simulink model "FIR_32tap"  (Simulink 7.0)
settings: Solver=FixedStepDiscrete  StartTime=0.0  StopTime=2048*sample_time  RelTol=1e-3
PreLoadFcn:
  | FIR_32tap_setup
InitFcn:
  | %% DSPBuilder Start
  | alt_dspbuilder_update_model(bdroot)
  | %% DSPBuilder End
undefined symbols (not defined in the file): fir_coeff, get, sample_time
libraries: allblocks_alteradspbuilder2 x43, dspsnks4 x2, Stratix_EP2S60_alteradspbuilder2 x2
settings Model: Creator=davlin  LastModifiedBy=davlin
settings DebuggingCC: SaveWithParameterizedLinksMsg=none
settings GRTTargetCC: TargetFcnLib=ansi_tfl_tmw.mat

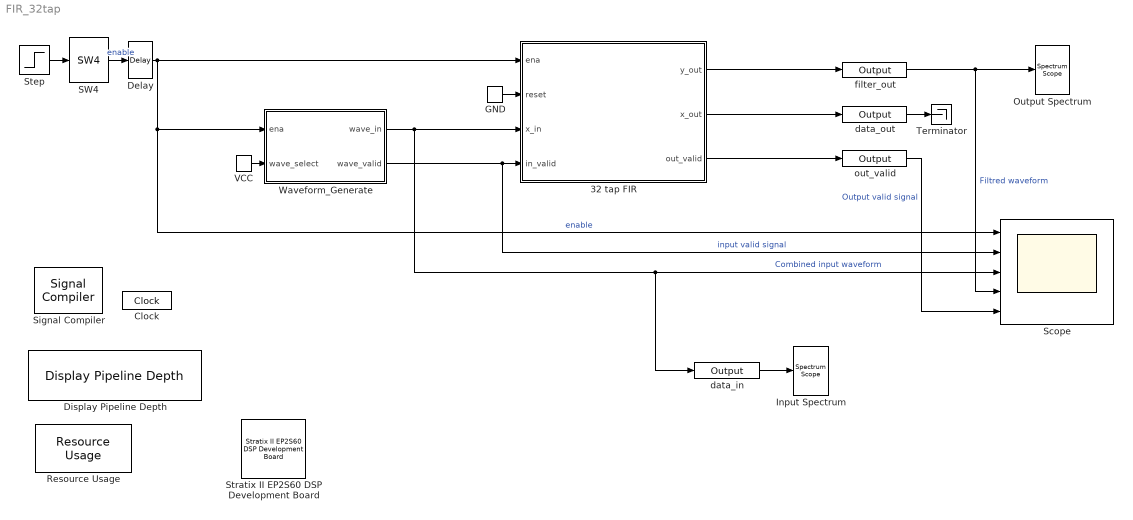
== system FIR_32tap ==
  32 tap FIR : Subsystem
  Clock : allblocks_alteradspbuilder2/Clock  ClockPeriod=clock_period  ClockPeriodUnit=ns  SampleTime=sample_time  SimulationStartCycle=5  PhaseOffset=0  Reset=aclr  ResetType=Active Low  Export=off
  Delay : allblocks_alteradspbuilder2/Delay  pipeline=1  pipeline_display=1  ClockPhase=1  use_ena=off  use_sclr=off  allowFloatingPointOverride=on  logOutputs=off  logFile=C:\Training\DSP_Training\Labs\DSPB_QII_V_9_0\Ex3\partc\tb_FIR_32tap\FIR%5F32tap_Delay.fixedpointlog  use_init=off  reset_value=1
  Display Pipeline Depth : allblocks_alteradspbuilder2/Display Pipeline Depth  DisplayLatencyOnBlocks=on
  GND : allblocks_alteradspbuilder2/GND  SpecifyClock=on  clock=Clock
  Input Spectrum : dspsnks4/Spectrum Scope  DialogController=dspdialog.SpectrumScope  DialogControllerArgs=DataTag0  SystemSampleTime=-1  ScopeProperties=on  Domain=Frequency  HorizSpan=1  UseBuffer=on  BufferSize=128  Overlap=64  inpFftLenInherit=off  FFTlength=128  numAvg=2  DisplayProperties=off  AxisGrid=on  Memory=off  FrameNumber=on  AxisLegend=off  AxisZoom=off  OpenScopeAtSimStart=on  OpenScopeImmediately=off  FigPos=get(0,'defaultfigureposition')  AxisProperties=off  XUnits=Hertz  XRange=[0...Fs/2]  InheritXIncr=on  XIncr=1.0  XLabel=Samples  XLimit=Auto  YUnits=dB  XMax=1  XMin=0  YLabel=Magnitude-squared, dB  LineProperties=off  wintypeSpecScope=Kaiser  RsSpecScope=50  betaSpecScope=5  winsampSpecScope=Periodic
      settings: YMin=1.0709621458062  YMax=69.4519012654706
  Output Spectrum : dspsnks4/Spectrum Scope  DialogController=dspdialog.SpectrumScope  DialogControllerArgs=DataTag1  SystemSampleTime=-1  ScopeProperties=on  Domain=Frequency  HorizSpan=1  UseBuffer=on  BufferSize=128  Overlap=64  inpFftLenInherit=off  FFTlength=128  numAvg=2  DisplayProperties=off  AxisGrid=on  Memory=off  FrameNumber=on  AxisLegend=off  AxisZoom=off  OpenScopeAtSimStart=on  OpenScopeImmediately=off  FigPos=get(0,'defaultfigureposition')  AxisProperties=off  XUnits=Hertz  XRange=[0...Fs/2]  InheritXIncr=on  XIncr=1.0  XLabel=Samples  XLimit=Auto  YUnits=dB  XMax=1  XMin=0  YLabel=Magnitude-squared, dB  LineProperties=off  wintypeSpecScope=Kaiser  RsSpecScope=50  betaSpecScope=5  winsampSpecScope=Periodic
      settings: YMin=-2.30591385737013  YMax=68.9595708716215
  Resource Usage : allblocks_alteradspbuilder2/Resource Usage  logic=3 %%  memory=< 1 %%  dsp=11 %%  memoryLable=Block RAM  dspLable=DSP
  SW4 : Stratix_EP2S60_alteradspbuilder2/SW4  iofile=C:\Training\DSP_Training\Labs\DSPB_QII_V_9_0\Ex3\partc\tb_FIR_32tap\FIR%5F32tap_SW4.salt  externalType=Inferred  SpecifyClock=on  clock=Clock  location=Pin_K14
  Scope : Scope  NumInputPorts=5
      settings: YMin=-500~-750~-1000~-750~-5  YMax=500~750~1000~750~5  Decimation=sample_time  SampleInput=on  SampleTime=sample_time
  Signal Compiler : allblocks_alteradspbuilder2/Signal Compiler  DeviceFamily=Stratix II  DeviceName=EP2S60F1020C4ES  EnableSignalTap=off  SignalTapDepth=256  UseBoardBlock=on  StpUseDefaultClock=on  StpClock=Clock  ExportDir=C:\Test\SR10650919
  Step : Step  Time=1*sample_time  SampleTime=sample_time
  Stratix II EP2S60 DSP Development Board : Stratix_EP2S60_alteradspbuilder2/Stratix II EP2S60 DSP Development Board  ClockPinIn=Pin_AM17  GlobalResetPin=Pin_AG19  device=EP2S60F1020C4ES
  Terminator : Terminator
  VCC : allblocks_alteradspbuilder2/VCC  SpecifyClock=off
  Waveform_Generate : Subsystem
  data_in : allblocks_alteradspbuilder2/Output  iofile=C:\Training\DSP_Training\Labs\DSPB_QII_V_9_0\Ex3\partc\tb_FIR_32tap\FIR%5F32tap_data%5Fin.capture  BusType=Signed Integer  bwl=12  bwr=0  externalType=Inferred  PORTTYPE=Output  allowFloatingPointOverride=on  logOutputs=off
  data_out : allblocks_alteradspbuilder2/Output  iofile=C:\Training\DSP_Training\Labs\DSPB_QII_V_9_0\Ex3\partc\tb_FIR_32tap\FIR%5F32tap_data%5Fout.capture  BusType=Signed Integer  bwl=12  bwr=0  externalType=Inferred  PORTTYPE=Output  allowFloatingPointOverride=on  logOutputs=off
  filter_out : allblocks_alteradspbuilder2/Output  iofile=C:\Training\DSP_Training\Labs\DSPB_QII_V_9_0\Ex3\partc\tb_FIR_32tap\FIR%5F32tap_filter%5Fout.capture  BusType=Signed Fractional  bwl=16  bwr=11  externalType=Inferred  PORTTYPE=Output  allowFloatingPointOverride=on  logOutputs=off
  out_valid : allblocks_alteradspbuilder2/Output  iofile=C:\Training\DSP_Training\Labs\DSPB_QII_V_9_0\Ex3\partc\tb_FIR_32tap\FIR%5F32tap_out%5Fvalid.capture  BusType=Single Bit  bwl=8  bwr=0  externalType=Inferred  PORTTYPE=Output  allowFloatingPointOverride=on  logOutputs=off
  wires:
  Step/1 -> SW4/1
  Waveform_Generate/2(wave_valid) -> Scope/2, 32 tap FIR/4(in_valid)  "input valid signal"
  32 tap FIR/1(y_out) -> filter_out/1
  32 tap FIR/2(x_out) -> data_out/1
  32 tap FIR/3(out_valid) -> out_valid/1
  GND/1 -> 32 tap FIR/2(reset)
  Waveform_Generate/1(wave_in) -> 32 tap FIR/3(x_in), Scope/3, data_in/1  "Combined input waveform"
  SW4/1 -> Delay/1  "enable"
  filter_out/1 -> Scope/4, Output Spectrum/1  "Filtred waveform"
  out_valid/1 -> Scope/5  "Output valid signal"
  data_in/1 -> Input Spectrum/1
  data_out/1 -> Terminator/1
  VCC/1 -> Waveform_Generate/2(wave_select)
  Delay/1 -> Scope/1, Waveform_Generate/1(ena), 32 tap FIR/1(ena)  "enable"

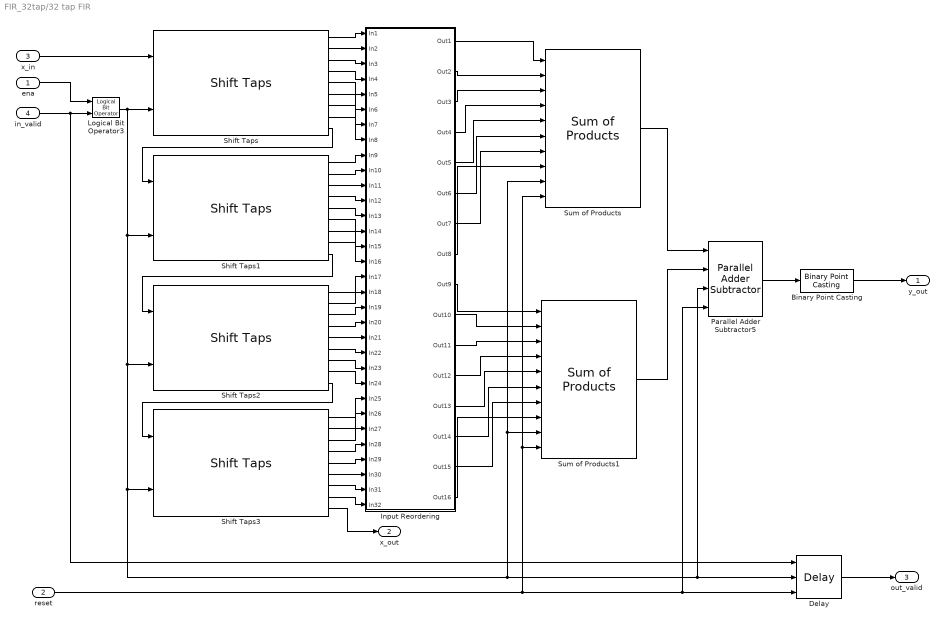
== system FIR_32tap/32 tap FIR ==
  ena : Inport  OutDataType=sfix(16)  OutScaling=2^0
  reset : Inport  Port=2  OutDataType=sfix(16)  OutScaling=2^0
  x_in : Inport  Port=3  OutDataType=sfix(16)  OutScaling=2^0
  in_valid : Inport  Port=4  OutDataType=sfix(16)  OutScaling=2^0
  Binary Point Casting : allblocks_alteradspbuilder2/Binary Point Casting  BusType=Signed Fractional  bwl=27  bwr=0  OutputPointPosition=11  pipeline_display=0
  Delay : allblocks_alteradspbuilder2/Delay  pipeline=35  pipeline_display=35  ClockPhase=1  use_ena=on  use_sclr=on  allowFloatingPointOverride=on  logOutputs=off  logFile=C:\Training\DSP_Training\Labs\DSPB_QII_V_9_0\Ex3\partc\tb_FIR_32tap\FIR%5F32tap_32+tap+FIR_Delay.fixedpointlog  use_init=off  reset_value=1
  Input Reordering : Subsystem  mask(Input Reordering - Custom Blocks){pipeline_level=1}
      mask prompts: pipeline_level "Pipeline Level:"
      mask help: This block reorders the output of the shift register.
  Logical Bit Operator3 : allblocks_alteradspbuilder2/Logical Bit Operator  LogicalOperator=AND  user_inputs=2  pipeline_display=0
  Parallel Adder Subtractor5 : allblocks_alteradspbuilder2/Parallel Adder Subtractor  number_of_inputs=2  direction=++  use_pipeline=on  pipeline_display=1  phase_selection=1  use_ena=on  use_aclr=on  allowFloatingPointOverride=on  logOutputs=off  logFile=C:\Training\DSP_Training\Labs\DSPB_QII_V_9_0\Ex3\partc\tb_FIR_32tap\FIR%5F32tap_32+tap+FIR_Parallel+Adder+Subtractor5.fixedpointlog
  Shift Taps : allblocks_alteradspbuilder2/Shift Taps  number_of_taps=8  tap_distance=1  use_shiftout=on  use_ena=on  use_sclr=off  use_dedicated_circuitry=on  ram_type=AUTO  allowFloatingPointOverride=on  logOutputs=off  logFile=C:\Training\DSP_Training\Labs\DSPB_QII_V_9_0\Ex3\partc\tb_FIR_32tap\FIR%5F32tap_32+tap+FIR_Shift+Taps%3A%3At.fixedpointlog,C:\Training\DSP_Training\Labs\DSPB_QII_V_9_0\Ex3\partc\tb_FIR_32tap\FIR%5F32tap_32+tap+FIR_Shift+Taps%3A%3At.fixedpointlog,C:\Training\DSP_Training\Labs\DSPB_QII_V_9_0\Ex3\partc\tb_FIR_32tap\FIR%5F32tap_32+tap+FIR_Shift+Taps%3A%3At.fixedpointlog,C:\Training\DSP_Training\Labs\DSPB_QII_V_9_0\Ex3\partc\tb_FIR_32tap\FIR%5F32tap_32+tap+FIR_Shift+Taps%3A%3At.fixedpointlog,C:\Training\DSP_Training\Labs\DSPB_QII_V_9_0\Ex3\partc\tb_FIR_32tap\FIR%5F32tap_32+tap+FIR_Shift+Taps%3A%3At.fixedpointlog,C:\Training\DSP_Training\Labs\DSPB_QII_V_9_0\Ex3\partc\tb_FIR_32tap\FIR%5F32tap_32+tap+FIR_Shift+Taps%3A%3At.fixedpointlog,C:\Training\DSP_Training\Labs\DSPB_QII_V_9_0\Ex3\partc\tb_FIR_32tap\FIR%5F32tap_32+tap+FIR_Shift+Taps%3A%3At.fixedpointlog,C:\Training\DSP_Training\Labs\DSPB_QII_V_9_0\Ex3\partc\tb_FIR_32tap\FIR%5F32tap_32+tap+FIR_Shift+Taps%3A%3At.fixedpointlog,C:\Training\DSP_Training\Labs\DSPB_QII_V_9_0\Ex3\partc\tb_FIR_32tap\FIR%5F32tap_32+tap+FIR_Shift+Taps%3A%3Ashiftout.fixedpointlog,
  Shift Taps1 : allblocks_alteradspbuilder2/Shift Taps  number_of_taps=8  tap_distance=1  use_shiftout=on  use_ena=on  use_sclr=off  use_dedicated_circuitry=on  ram_type=AUTO  allowFloatingPointOverride=on  logOutputs=off  logFile=C:\Training\DSP_Training\Labs\DSPB_QII_V_9_0\Ex3\partc\tb_FIR_32tap\FIR%5F32tap_32+tap+FIR_Shift+Taps1%3A%3At.fixedpointlog,C:\Training\DSP_Training\Labs\DSPB_QII_V_9_0\Ex3\partc\tb_FIR_32tap\FIR%5F32tap_32+tap+FIR_Shift+Taps1%3A%3At.fixedpointlog,C:\Training\DSP_Training\Labs\DSPB_QII_V_9_0\Ex3\partc\tb_FIR_32tap\FIR%5F32tap_32+tap+FIR_Shift+Taps1%3A%3At.fixedpointlog,C:\Training\DSP_Training\Labs\DSPB_QII_V_9_0\Ex3\partc\tb_FIR_32tap\FIR%5F32tap_32+tap+FIR_Shift+Taps1%3A%3At.fixedpointlog,C:\Training\DSP_Training\Labs\DSPB_QII_V_9_0\Ex3\partc\tb_FIR_32tap\FIR%5F32tap_32+tap+FIR_Shift+Taps1%3A%3At.fixedpointlog,C:\Training\DSP_Training\Labs\DSPB_QII_V_9_0\Ex3\partc\tb_FIR_32tap\FIR%5F32tap_32+tap+FIR_Shift+Taps1%3A%3At.fixedpointlog,C:\Training\DSP_Training\Labs\DSPB_QII_V_9_0\Ex3\partc\tb_FIR_32tap\FIR%5F32tap_32+tap+FIR_Shift+Taps1%3A%3At.fixedpointlog,C:\Training\DSP_Training\Labs\DSPB_QII_V_9_0\Ex3\partc\tb_FIR_32tap\FIR%5F32tap_32+tap+FIR_Shift+Taps1%3A%3At.fixedpointlog,C:\Training\DSP_Training\Labs\DSPB_QII_V_9_0\Ex3\partc\tb_FIR_32tap\FIR%5F32tap_32+tap+FIR_Shift+Taps1%3A%3Ashiftout.fixedpointlog,
  Shift Taps2 : allblocks_alteradspbuilder2/Shift Taps  number_of_taps=8  tap_distance=1  use_shiftout=on  use_ena=on  use_sclr=off  use_dedicated_circuitry=on  ram_type=AUTO  allowFloatingPointOverride=on  logOutputs=off  logFile=C:\Training\DSP_Training\Labs\DSPB_QII_V_9_0\Ex3\partc\tb_FIR_32tap\FIR%5F32tap_32+tap+FIR_Shift+Taps2%3A%3At.fixedpointlog,C:\Training\DSP_Training\Labs\DSPB_QII_V_9_0\Ex3\partc\tb_FIR_32tap\FIR%5F32tap_32+tap+FIR_Shift+Taps2%3A%3At.fixedpointlog,C:\Training\DSP_Training\Labs\DSPB_QII_V_9_0\Ex3\partc\tb_FIR_32tap\FIR%5F32tap_32+tap+FIR_Shift+Taps2%3A%3At.fixedpointlog,C:\Training\DSP_Training\Labs\DSPB_QII_V_9_0\Ex3\partc\tb_FIR_32tap\FIR%5F32tap_32+tap+FIR_Shift+Taps2%3A%3At.fixedpointlog,C:\Training\DSP_Training\Labs\DSPB_QII_V_9_0\Ex3\partc\tb_FIR_32tap\FIR%5F32tap_32+tap+FIR_Shift+Taps2%3A%3At.fixedpointlog,C:\Training\DSP_Training\Labs\DSPB_QII_V_9_0\Ex3\partc\tb_FIR_32tap\FIR%5F32tap_32+tap+FIR_Shift+Taps2%3A%3At.fixedpointlog,C:\Training\DSP_Training\Labs\DSPB_QII_V_9_0\Ex3\partc\tb_FIR_32tap\FIR%5F32tap_32+tap+FIR_Shift+Taps2%3A%3At.fixedpointlog,C:\Training\DSP_Training\Labs\DSPB_QII_V_9_0\Ex3\partc\tb_FIR_32tap\FIR%5F32tap_32+tap+FIR_Shift+Taps2%3A%3At.fixedpointlog,C:\Training\DSP_Training\Labs\DSPB_QII_V_9_0\Ex3\partc\tb_FIR_32tap\FIR%5F32tap_32+tap+FIR_Shift+Taps2%3A%3Ashiftout.fixedpointlog,
  Shift Taps3 : allblocks_alteradspbuilder2/Shift Taps  number_of_taps=8  tap_distance=1  use_shiftout=on  use_ena=on  use_sclr=off  use_dedicated_circuitry=on  ram_type=AUTO  allowFloatingPointOverride=on  logOutputs=off  logFile=C:\Training\DSP_Training\Labs\DSPB_QII_V_9_0\Ex3\partc\tb_FIR_32tap\FIR%5F32tap_32+tap+FIR_Shift+Taps3%3A%3At.fixedpointlog,C:\Training\DSP_Training\Labs\DSPB_QII_V_9_0\Ex3\partc\tb_FIR_32tap\FIR%5F32tap_32+tap+FIR_Shift+Taps3%3A%3At.fixedpointlog,C:\Training\DSP_Training\Labs\DSPB_QII_V_9_0\Ex3\partc\tb_FIR_32tap\FIR%5F32tap_32+tap+FIR_Shift+Taps3%3A%3At.fixedpointlog,C:\Training\DSP_Training\Labs\DSPB_QII_V_9_0\Ex3\partc\tb_FIR_32tap\FIR%5F32tap_32+tap+FIR_Shift+Taps3%3A%3At.fixedpointlog,C:\Training\DSP_Training\Labs\DSPB_QII_V_9_0\Ex3\partc\tb_FIR_32tap\FIR%5F32tap_32+tap+FIR_Shift+Taps3%3A%3At.fixedpointlog,C:\Training\DSP_Training\Labs\DSPB_QII_V_9_0\Ex3\partc\tb_FIR_32tap\FIR%5F32tap_32+tap+FIR_Shift+Taps3%3A%3At.fixedpointlog,C:\Training\DSP_Training\Labs\DSPB_QII_V_9_0\Ex3\partc\tb_FIR_32tap\FIR%5F32tap_32+tap+FIR_Shift+Taps3%3A%3At.fixedpointlog,C:\Training\DSP_Training\Labs\DSPB_QII_V_9_0\Ex3\partc\tb_FIR_32tap\FIR%5F32tap_32+tap+FIR_Shift+Taps3%3A%3At.fixedpointlog,C:\Training\DSP_Training\Labs\DSPB_QII_V_9_0\Ex3\partc\tb_FIR_32tap\FIR%5F32tap_32+tap+FIR_Shift+Taps3%3A%3Ashiftout.fixedpointlog,
  Sum of Products : allblocks_alteradspbuilder2/Sum of Products  BusType=Signed Integer  InputBwl=12  InputBwr=0  number_of_coefficients=8  CoefBwl=12  CoefBwr=0  coefficients=fir_coeff(1:8)  pipeline=1  pipeline_display=1  full_resolution=on  OutputBwl=8  OutputBwr=0  TruncateLsb=0  implementation=Dedicated Multiplier Circuitry  use_ena=on  use_aclr=on
  Sum of Products1 : allblocks_alteradspbuilder2/Sum of Products  BusType=Signed Integer  InputBwl=12  InputBwr=0  number_of_coefficients=8  CoefBwl=12  CoefBwr=0  coefficients=fir_coeff(9:16)  pipeline=1  pipeline_display=1  full_resolution=on  OutputBwl=8  OutputBwr=0  TruncateLsb=0  implementation=Dedicated Multiplier Circuitry  use_ena=on  use_aclr=on
  y_out : Outport  OutDataType=sfix(16)  OutScaling=2^0
  x_out : Outport  Port=2  OutDataType=sfix(16)  OutScaling=2^0
  out_valid : Outport  Port=3  OutDataType=sfix(16)  OutScaling=2^0
  wires:
  Delay/1 -> out_valid/1
  reset/1 -> Sum of Products/10, Sum of Products1/10, Delay/3, Parallel Adder Subtractor5/4
  x_in/1 -> Shift Taps/1
  Shift Taps2/9 -> Shift Taps3/1
  Logical Bit Operator3/1 -> Shift Taps/2, Shift Taps1/2, Shift Taps2/2, Shift Taps3/2, Delay/2, Parallel Adder Subtractor5/3, Sum of Products1/9, Sum of Products/9
  Shift Taps/9 -> Shift Taps1/1
  Shift Taps1/9 -> Shift Taps2/1
  Shift Taps/1 -> Input Reordering/1(In1)
  Shift Taps/2 -> Input Reordering/2(In2)
  Shift Taps/3 -> Input Reordering/3(In3)
  Shift Taps/4 -> Input Reordering/4(In4)
  Shift Taps/5 -> Input Reordering/5(In5)
  Shift Taps/6 -> Input Reordering/6(In6)
  Shift Taps/7 -> Input Reordering/7(In7)
  Shift Taps/8 -> Input Reordering/8(In8)
  Shift Taps1/1 -> Input Reordering/9(In9)
  Shift Taps1/2 -> Input Reordering/10(In10)
  Shift Taps1/3 -> Input Reordering/11(In11)
  Shift Taps1/4 -> Input Reordering/12(In12)
  Shift Taps1/5 -> Input Reordering/13(In13)
  Shift Taps1/6 -> Input Reordering/14(In14)
  Shift Taps1/7 -> Input Reordering/15(In15)
  Shift Taps1/8 -> Input Reordering/16(In16)
  Shift Taps2/1 -> Input Reordering/17(In17)
  Shift Taps2/2 -> Input Reordering/18(In18)
  Shift Taps2/3 -> Input Reordering/19(In19)
  Shift Taps2/4 -> Input Reordering/20(In20)
  Shift Taps2/5 -> Input Reordering/21(In21)
  Shift Taps2/6 -> Input Reordering/22(In22)
  Shift Taps2/7 -> Input Reordering/23(In23)
  Shift Taps2/8 -> Input Reordering/24(In24)
  Shift Taps3/1 -> Input Reordering/25(In25)
  Shift Taps3/2 -> Input Reordering/26(In26)
  Shift Taps3/3 -> Input Reordering/27(In27)
  Shift Taps3/4 -> Input Reordering/28(In28)
  Shift Taps3/5 -> Input Reordering/29(In29)
  Shift Taps3/6 -> Input Reordering/30(In30)
  Shift Taps3/7 -> Input Reordering/31(In31)
  Shift Taps3/8 -> Input Reordering/32(In32)
  Input Reordering/1(Out1) -> Sum of Products/1
  Input Reordering/2(Out2) -> Sum of Products/2
  Input Reordering/3(Out3) -> Sum of Products/3
  Input Reordering/9(Out9) -> Sum of Products1/1
  Input Reordering/10(Out10) -> Sum of Products1/2
  Input Reordering/11(Out11) -> Sum of Products1/3
  Input Reordering/12(Out12) -> Sum of Products1/4
  Input Reordering/13(Out13) -> Sum of Products1/5
  Input Reordering/14(Out14) -> Sum of Products1/6
  Input Reordering/15(Out15) -> Sum of Products1/7
  Input Reordering/16(Out16) -> Sum of Products1/8
  in_valid/1 -> Logical Bit Operator3/2, Delay/1
  ena/1 -> Logical Bit Operator3/1
  Sum of Products/1 -> Parallel Adder Subtractor5/1
  Sum of Products1/1 -> Parallel Adder Subtractor5/2
  Parallel Adder Subtractor5/1 -> Binary Point Casting/1
  Shift Taps3/9 -> x_out/1
  Input Reordering/4(Out4) -> Sum of Products/4
  Input Reordering/5(Out5) -> Sum of Products/5
  Input Reordering/6(Out6) -> Sum of Products/6
  Input Reordering/7(Out7) -> Sum of Products/7
  Input Reordering/8(Out8) -> Sum of Products/8
  Binary Point Casting/1 -> y_out/1

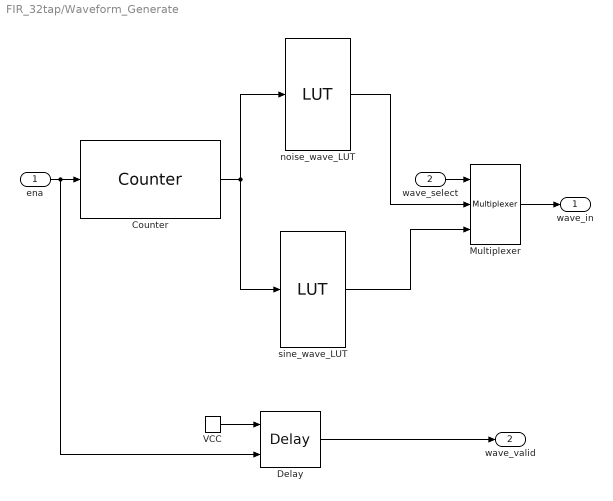
== system FIR_32tap/Waveform_Generate ==
  ena : Inport  OutDataType=sfix(16)  OutScaling=2^0
  wave_select : Inport  Port=2  OutDataType=sfix(16)  OutScaling=2^0
  Counter : allblocks_alteradspbuilder2/Counter  BusType=Unsigned Integer  bwl=10  bwr=0  use_modulo=on  modulo=900  SpecifyClock=on  clock=Clock  direction=Increment  use_sload=off  use_sset=off  svalue=1  use_clk_ena=off  use_ena=on  use_sclr=off  pipeline_display=1
  Delay : allblocks_alteradspbuilder2/Delay  pipeline=2  pipeline_display=2  ClockPhase=1  use_ena=on  use_sclr=off  allowFloatingPointOverride=on  logOutputs=off  logFile=C:\Training\DSP_Training\Labs\DSPB_QII_V_9_0\Ex3\partc\tb_FIR_32tap\FIR%5F32tap_Waveform%5FGenerate_Delay.fixedpointlog  use_init=off  reset_value=1
  Multiplexer : allblocks_alteradspbuilder2/Multiplexer  numInputs=2  pipeline=0  oneHot=off  pipeline_display=0  use_ena=off  use_aclr=off  allowFloatingPointOverride=on  logOutputs=off  logFile=C:\Training\DSP_Training\Labs\DSPB_QII_V_9_0\Ex3\partc\tb_FIR_32tap\FIR%5F32tap_Waveform%5FGenerate_Multiplexer.fixedpointlog
  VCC : allblocks_alteradspbuilder2/VCC  SpecifyClock=on  clock=Clock
  noise_wave_LUT : allblocks_alteradspbuilder2/LUT  addr_width=10  BusType=Signed Integer  bwl=12  bwr=0  init_array=noise_in  allowFloatingPointOverride=on  logOutputs=off  logFile=C:\Training\DSP_Training\Labs\DSPB_QII_V_9_0\Ex3\partc\tb_FIR_32tap\FIR%5F32tap_Waveform%5FGenerate_noise%5Fwave%5FLUT.fixedpointlog  use_ena=off  reg_data=off  use_lpm=on  reg_addr=on  ram_type=AUTO  pipeline_display=1
  sine_wave_LUT : allblocks_alteradspbuilder2/LUT  addr_width=10  BusType=Signed Integer  bwl=12  bwr=0  init_array=sine_in  allowFloatingPointOverride=on  logOutputs=off  logFile=C:\Training\DSP_Training\Labs\DSPB_QII_V_9_0\Ex3\partc\tb_FIR_32tap\FIR%5F32tap_Waveform%5FGenerate_sine%5Fwave%5FLUT.fixedpointlog  use_ena=off  reg_data=off  use_lpm=on  reg_addr=on  ram_type=AUTO  pipeline_display=1
  wave_in : Outport  OutDataType=sfix(16)  OutScaling=2^0
  wave_valid : Outport  Port=2  OutDataType=sfix(16)  OutScaling=2^0
  wires:
  wave_select/1 -> Multiplexer/1
  ena/1 -> Delay/2, Counter/1
  Multiplexer/1 -> wave_in/1
  VCC/1 -> Delay/1
  Delay/1 -> wave_valid/1
  sine_wave_LUT/1 -> Multiplexer/3
  noise_wave_LUT/1 -> Multiplexer/2
  Counter/1 -> noise_wave_LUT/1, sine_wave_LUT/1

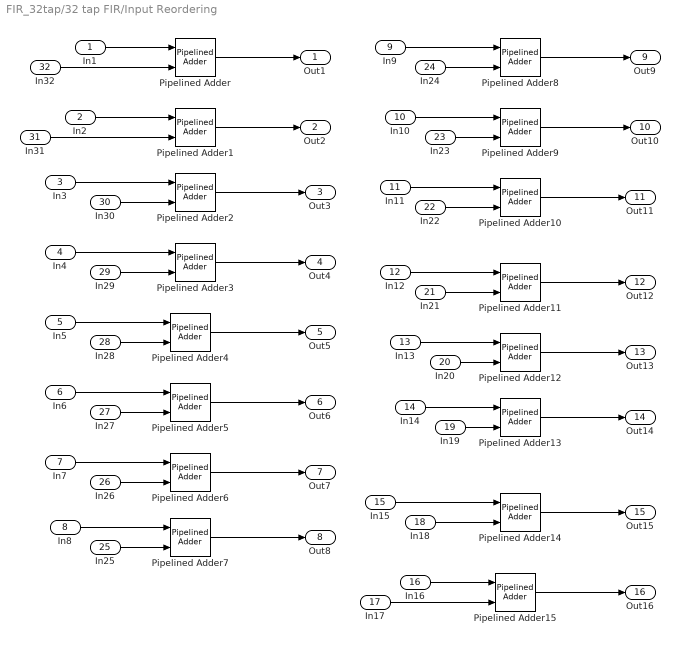
== system FIR_32tap/32 tap FIR/Input Reordering ==
  In1 : Inport  OutDataType=sfix(16)  OutScaling=2^0
  In2 : Inport  Port=2  OutDataType=sfix(16)  OutScaling=2^0
  In3 : Inport  Port=3  OutDataType=sfix(16)  OutScaling=2^0
  In4 : Inport  Port=4  OutDataType=sfix(16)  OutScaling=2^0
  In5 : Inport  Port=5  OutDataType=sfix(16)  OutScaling=2^0
  In6 : Inport  Port=6  OutDataType=sfix(16)  OutScaling=2^0
  In7 : Inport  Port=7  OutDataType=sfix(16)  OutScaling=2^0
  In8 : Inport  Port=8  OutDataType=sfix(16)  OutScaling=2^0
  In9 : Inport  Port=9  OutDataType=sfix(16)  OutScaling=2^0
  In10 : Inport  Port=10  OutDataType=sfix(16)  OutScaling=2^0
  In11 : Inport  Port=11  OutDataType=sfix(16)  OutScaling=2^0
  In12 : Inport  Port=12  OutDataType=sfix(16)  OutScaling=2^0
  In13 : Inport  Port=13  OutDataType=sfix(16)  OutScaling=2^0
  In14 : Inport  Port=14  OutDataType=sfix(16)  OutScaling=2^0
  In15 : Inport  Port=15  OutDataType=sfix(16)  OutScaling=2^0
  In16 : Inport  Port=16  OutDataType=sfix(16)  OutScaling=2^0
  In17 : Inport  Port=17  OutDataType=sfix(16)  OutScaling=2^0
  In18 : Inport  Port=18  OutDataType=sfix(16)  OutScaling=2^0
  In19 : Inport  Port=19  OutDataType=sfix(16)  OutScaling=2^0
  In20 : Inport  Port=20  OutDataType=sfix(16)  OutScaling=2^0
  In21 : Inport  Port=21  OutDataType=sfix(16)  OutScaling=2^0
  In22 : Inport  Port=22  OutDataType=sfix(16)  OutScaling=2^0
  In23 : Inport  Port=23  OutDataType=sfix(16)  OutScaling=2^0
  In24 : Inport  Port=24  OutDataType=sfix(16)  OutScaling=2^0
  In25 : Inport  Port=25  OutDataType=sfix(16)  OutScaling=2^0
  In26 : Inport  Port=26  OutDataType=sfix(16)  OutScaling=2^0
  In27 : Inport  Port=27  OutDataType=sfix(16)  OutScaling=2^0
  In28 : Inport  Port=28  OutDataType=sfix(16)  OutScaling=2^0
  In29 : Inport  Port=29  OutDataType=sfix(16)  OutScaling=2^0
  In30 : Inport  Port=30  OutDataType=sfix(16)  OutScaling=2^0
  In31 : Inport  Port=31  OutDataType=sfix(16)  OutScaling=2^0
  In32 : Inport  Port=32  OutDataType=sfix(16)  OutScaling=2^0
  Pipelined Adder{,1..15} (16 alike) : allblocks_alteradspbuilder2/Pipelined Adder  BusType=Signed Integer  bwl=12  bwr=0  pipeline=pipeline_level  pipeline_display=0  AddSubDirection=ADD  use_cin=off  use_ovl=off  use_addsub=off  use_ena=off  use_aclr=off
  Out1 : Outport  OutDataType=sfix(16)  OutScaling=2^0
  Out2 : Outport  Port=2  OutDataType=sfix(16)  OutScaling=2^0
  Out3 : Outport  Port=3  OutDataType=sfix(16)  OutScaling=2^0
  Out4 : Outport  Port=4  OutDataType=sfix(16)  OutScaling=2^0
  Out5 : Outport  Port=5  OutDataType=sfix(16)  OutScaling=2^0
  Out6 : Outport  Port=6  OutDataType=sfix(16)  OutScaling=2^0
  Out7 : Outport  Port=7  OutDataType=sfix(16)  OutScaling=2^0
  Out8 : Outport  Port=8  OutDataType=sfix(16)  OutScaling=2^0
  Out9 : Outport  Port=9  OutDataType=sfix(16)  OutScaling=2^0
  Out10 : Outport  Port=10  OutDataType=sfix(16)  OutScaling=2^0
  Out11 : Outport  Port=11  OutDataType=sfix(16)  OutScaling=2^0
  Out12 : Outport  Port=12  OutDataType=sfix(16)  OutScaling=2^0
  Out13 : Outport  Port=13  OutDataType=sfix(16)  OutScaling=2^0
  Out14 : Outport  Port=14  OutDataType=sfix(16)  OutScaling=2^0
  Out15 : Outport  Port=15  OutDataType=sfix(16)  OutScaling=2^0
  Out16 : Outport  Port=16  OutDataType=sfix(16)  OutScaling=2^0
  wires:
  In1/1 -> Pipelined Adder/1
  In32/1 -> Pipelined Adder/2
  In2/1 -> Pipelined Adder1/1
  In31/1 -> Pipelined Adder1/2
  In3/1 -> Pipelined Adder2/1
  In4/1 -> Pipelined Adder3/1
  In5/1 -> Pipelined Adder4/1
  In6/1 -> Pipelined Adder5/1
  In7/1 -> Pipelined Adder6/1
  In8/1 -> Pipelined Adder7/1
  In9/1 -> Pipelined Adder8/1
  In11/1 -> Pipelined Adder10/1
  In12/1 -> Pipelined Adder11/1
  In13/1 -> Pipelined Adder12/1
  In14/1 -> Pipelined Adder13/1
  In15/1 -> Pipelined Adder14/1
  In10/1 -> Pipelined Adder9/1
  In16/1 -> Pipelined Adder15/1
  In17/1 -> Pipelined Adder15/2
  In18/1 -> Pipelined Adder14/2
  In19/1 -> Pipelined Adder13/2
  In20/1 -> Pipelined Adder12/2
  In21/1 -> Pipelined Adder11/2
  In22/1 -> Pipelined Adder10/2
  In23/1 -> Pipelined Adder9/2
  In24/1 -> Pipelined Adder8/2
  In25/1 -> Pipelined Adder7/2
  In26/1 -> Pipelined Adder6/2
  In27/1 -> Pipelined Adder5/2
  In28/1 -> Pipelined Adder4/2
  In29/1 -> Pipelined Adder3/2
  In30/1 -> Pipelined Adder2/2
  Pipelined Adder/1 -> Out1/1
  Pipelined Adder1/1 -> Out2/1
  Pipelined Adder2/1 -> Out3/1
  Pipelined Adder3/1 -> Out4/1
  Pipelined Adder4/1 -> Out5/1
  Pipelined Adder5/1 -> Out6/1
  Pipelined Adder6/1 -> Out7/1
  Pipelined Adder7/1 -> Out8/1
  Pipelined Adder8/1 -> Out9/1
  Pipelined Adder9/1 -> Out10/1
  Pipelined Adder10/1 -> Out11/1
  Pipelined Adder15/1 -> Out16/1
  Pipelined Adder14/1 -> Out15/1
  Pipelined Adder13/1 -> Out14/1
  Pipelined Adder12/1 -> Out13/1
  Pipelined Adder11/1 -> Out12/1
